simulink model "Junctions5_2018a"  (R2018a)
settings: Solver=VariableStepAuto  StartTime=0.0  StopTime=0.1  RelTol=1e-3
settings Model: Creator=BEAR  LastModifiedBy=bzhan

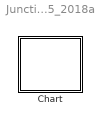
== system Junctions5_2018a ==
  Chart : Stateflow chart  TreatAsAtomicUnit=on

== stateflow chart Junctions5_2018a/Chart ==
  settings: updateMethod=DISCRETE  sampleTime=0.1
  state A
    en:f("enA")
    du:f("duA")
    ex:f("exA")
    state A1
      en:f("enA1")
      ex:f("exA1")
    state A2
      en: f("enA2")
    (default) -> A1
    A1 -> (junction 16)
    (junction 16) -> A2 [order 2]
  state C
    en:f("enC")
    ex:f("exC")
    state C1
      en:f("enC1")
    (default) -> C1
    (junction 19) -> C1 : [x<0]
  (default) -> A : {x=1;}
  (junction 16) -> (junction 19) [order 1] : {f("ca")}/{f("ta")}
  data: s function_input; x local
  function f(s):
    | function f(s)
    |     fprintf(s+"\n");
